simulink model "Integrator_extX0_verif"  (Simulink 7.2)
settings: Solver=ode45  StartTime=0.0  StopTime=10.0  RelTol=1e-3
undefined symbols (not defined in the file): integrator_sample
settings Model: Creator=Romain  LastModifiedBy=Romain
settings OptimizationCC: ExpressionDepthLimit=128
settings DebuggingCC: SolverPrmCheckMsg=none  FcnCallInpInsideContextMsg=Enable All  StateNameClashWarn=none  StrictBusMsg=ErrorLevel1
settings CodeAppCC: CustomSymbolStrType=$N$R$M_T
settings GRTTargetCC: TargetFunctionLibrary=C89/C90 (ANSI)

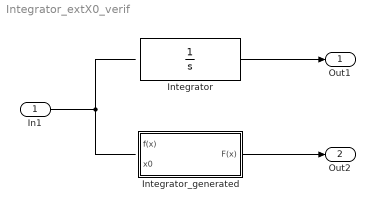
== system Integrator_extX0_verif ==
  In1 : Inport  OutDataTypeStr=double  DataType=double
  Integrator : Integrator  InitialConditionSource=external
  Integrator_generated : Subsystem  TreatAsAtomicUnit=on
  Out1 : Outport
  Out2 : Outport  Port=2
  wires:
  In1/1 -> ?
  Integrator/1 -> Out1/1
  Integrator_generated/1(F(x)) -> Out2/1

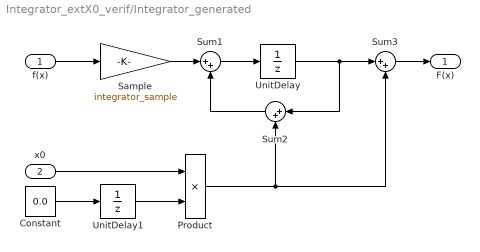
== system Integrator_extX0_verif/Integrator_generated ==
  f(x) : Inport
  x0 : Inport  Port=2
  Constant : Constant  Value=0.0  SampleTime=integrator_sample
  Product : Product  RndMeth=Zero
  Sample : Gain  Gain=integrator_sample
  Sum1 : Sum  RequirementInfo={} %GIDa_c455c9c0_ee5d_472b_80a9_71493720ee37  Inputs=|++
  Sum2 : Sum  RequirementInfo={} %GIDa_10f843ac_8bb4_4e78_8fd4_eab6d46ec7d5  Orientation=left  Inputs=|++
  Sum3 : Sum  RequirementInfo={} %GIDa_eff0dc0a_8709_422e_870a_136bf13f6bdf  Inputs=|++
  UnitDelay : UnitDelay  SampleTime=integrator_sample
  UnitDelay1 : UnitDelay  X0=1  SampleTime=integrator_sample
  F(x) : Outport  RequirementInfo={} %GIDa_b3b1b066_3038_423c_8101_59d6a2cdfb2b
  wires:
  Sum1/1 -> UnitDelay/1
  Sample/1 -> Sum1/1
  UnitDelay/1 -> Sum3/1, Sum2/1
  Sum2/1 -> Sum1/2
  Product/1 -> Sum3/2, Sum2/2
  UnitDelay1/1 -> Product/2
  Constant/1 -> UnitDelay1/1
  f(x)/1 -> Sample/1
  x0/1 -> Product/1
  Sum3/1 -> F(x)/1
